simulink model "feeder_1_2_sc_lh3"  (Simulink 9.2)
settings: Solver=ode4  StartTime=0.0  StopTime=inf  FixedStep=0.0001  RelTol=1e-3
PreLoadFcn:
  | Ts=100e-6;Core_Num = 0;
PostLoadFcn:
  | Ts=100e-6;Core_Num = 0;
InitFcn:
  | Ts=100e-6;Core_Num = 0;
libraries: opal_lib x1
settings Model: ARTEMISmethode_block_infos=$$__separator__$$  Creator=DETLDAQ  LastModifiedBy=DETLDAQ
settings OptimizationCC: BlockReduction=off  BooleanDataType=off  OptimizeBlockIOStorage=off  BufferReuse=off  GlobalBufferReuse=off  ExpressionFolding=off  LocalBlockOutputs=off  OptimizeDataStoreBuffers=off  BusAssignmentInplaceUpdate=off
settings DebuggingCC: SaveWithParameterizedLinksMsg=none  SignalResolutionControl=TryResolveAllWithWarning  MultiTaskDSMMsg=warning  MultiTaskCondExecSysMsg=none  FcnCallInpInsideContextMsg=error
settings HardwareCC: TargetUnknown=on
settings RTWCC: GenCodeOnly=on
settings GRTTargetCC: CombineOutputUpdateFcns=on  GRTInterface=off
settings SimscapeCC: SimscapeNormalizeSystem=off

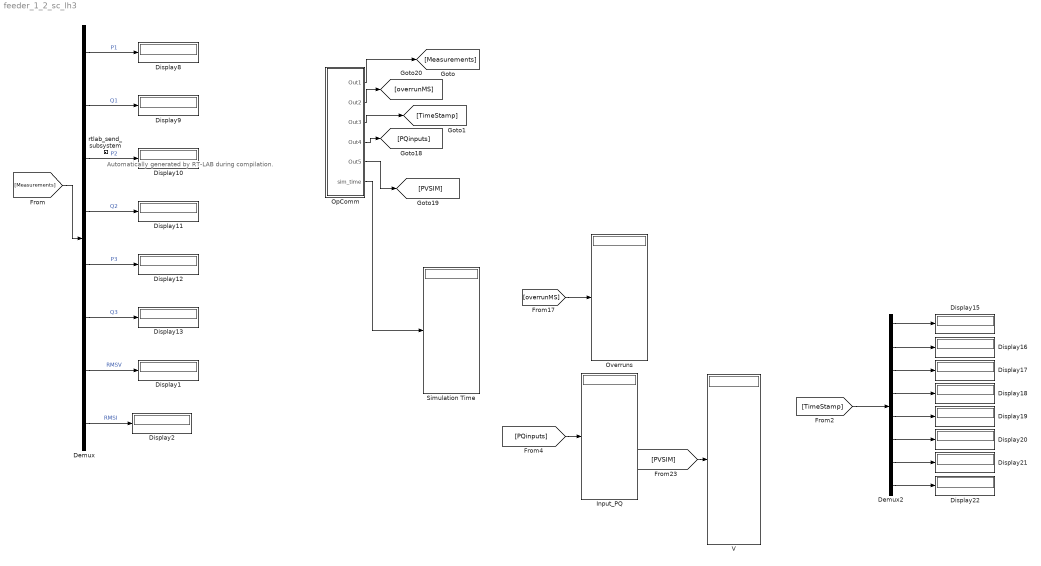
== system feeder_1_2_sc_lh3 ==
  note: Automatically generated by RT-LAB during compilation.
  Demux : Demux  Outputs=8
  Demux2 : Demux  Outputs=8
  Display{1..2,8..13,15..22} (16 alike) : Display
  Input_PQ : Display
  OpComm : Subsystem
      mask init:
      | opmaskdisplay('maskdisplay_block',gcb,'disp(''OpComm'')');
      mask Display:
      | patch([0 0.5 0.7 0],[1 1 0 0],[0.7 0.75 0.9]);
      | patch([1 0.53 0.73 1],[1 1 0 0],[1 0.8 0.7]);
      | plot([0 0 1 1 0],[0 1 1 0 0]);
      | disp('OpComm')
  Overruns : Display
  Simulation Time : Display
  V : Display
  rtlab_send_subsystem : Subsystem  Priority=-100
      mask Display: text(0,0,'');
  wires:
  Demux/7 -> Display1/1  "RMSV"
  Demux/8 -> Display2/1  "RMSI"
  OpComm/6(sim_time) -> Simulation Time/1
  OpComm/5(Out5) -> [PVSIM]
  OpComm/4(Out4) -> [PQinputs]
  [PQinputs] -> Input_PQ/1
  [PVSIM] -> V/1
  OpComm/3(Out3) -> [TimeStamp]
  OpComm/2(Out2) -> [overrunMS]
  OpComm/1(Out1) -> [Measurements]
  [overrunMS] -> Overruns/1
  Demux2/8 -> Display22/1
  Demux2/7 -> Display21/1
  Demux2/6 -> Display20/1
  Demux2/5 -> Display19/1
  Demux2/4 -> Display18/1
  Demux2/3 -> Display17/1
  Demux2/2 -> Display16/1
  Demux2/1 -> Display15/1
  [TimeStamp] -> Demux2/1
  [Measurements] -> Demux/1
  Demux/1 -> Display8/1  "P1"
  Demux/2 -> Display9/1  "Q1"
  Demux/3 -> Display10/1  "P2"
  Demux/4 -> Display11/1  "Q2"
  Demux/5 -> Display12/1  "P3"
  Demux/6 -> Display13/1  "Q3"

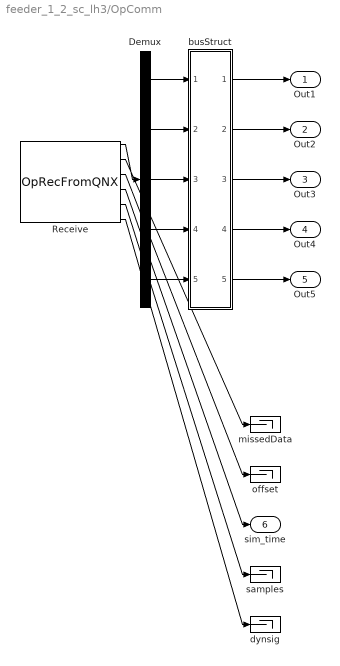
== system feeder_1_2_sc_lh3/OpComm ==
  Demux : Demux  Outputs="[8   1   8   6  12]"
  Receive : opal_lib/Communication/OpRecFromQNX  Node_num=1  Acqu_Group=1  Data_Width=35  Synchronization=on  Interpolation=on  Threshold=1.0  modelname=Feeder_1.mdl  sampletime=0.0001
  busStruct : Subsystem
  dynsig : Terminator
  missedData : Terminator
  offset : Terminator
  samples : Terminator
  Out1 : Outport
  Out2 : Outport  Port=2
  Out3 : Outport  Port=3
  Out4 : Outport  Port=4
  Out5 : Outport  Port=5
  sim_time : Outport  Port=6
  wires:
  Demux/5 -> busStruct/5(In5)
  Demux/4 -> busStruct/4(In4)
  Demux/3 -> busStruct/3(In3)
  Demux/2 -> busStruct/2(In2)
  Demux/1 -> busStruct/1(In1)
  busStruct/5(Out5) -> Out5/1
  busStruct/4(Out4) -> Out4/1
  busStruct/3(Out3) -> Out3/1
  busStruct/2(Out2) -> Out2/1
  busStruct/1(Out1) -> Out1/1
  Receive/1 -> Demux/1
  Receive/6 -> dynsig/1
  Receive/5 -> samples/1
  Receive/4 -> sim_time/1
  Receive/3 -> offset/1
  Receive/2 -> missedData/1

== system feeder_1_2_sc_lh3/rtlab_send_subsystem ==

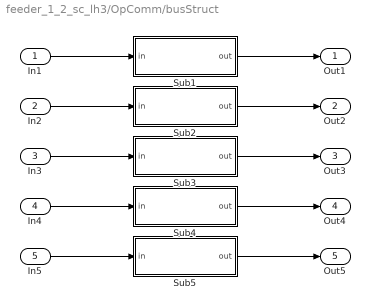
== system feeder_1_2_sc_lh3/OpComm/busStruct ==
  In1 : Inport
  In2 : Inport  Port=2
  In3 : Inport  Port=3
  In4 : Inport  Port=4
  In5 : Inport  Port=5
  Sub1 : Subsystem
  Sub2 : Subsystem
  Sub3 : Subsystem
  Sub4 : Subsystem
  Sub5 : Subsystem
  Out1 : Outport
  Out2 : Outport  Port=2
  Out3 : Outport  Port=3
  Out4 : Outport  Port=4
  Out5 : Outport  Port=5
  wires:
  Sub5/1(out) -> Out5/1
  In5/1 -> Sub5/1(in)
  Sub4/1(out) -> Out4/1
  In4/1 -> Sub4/1(in)
  Sub3/1(out) -> Out3/1
  In3/1 -> Sub3/1(in)
  Sub2/1(out) -> Out2/1
  In2/1 -> Sub2/1(in)
  Sub1/1(out) -> Out1/1
  In1/1 -> Sub1/1(in)

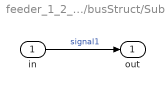
== system feeder_1_2_sc_lh3/OpComm/busStruct/Sub1 ==
  in : Inport
  out : Outport
  wires:
  in/1 -> out/1  "signal1"

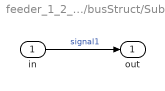
== system feeder_1_2_sc_lh3/OpComm/busStruct/Sub2 ==
  in : Inport
  out : Outport
  wires:
  in/1 -> out/1  "signal1"

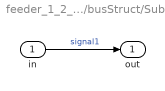
== system feeder_1_2_sc_lh3/OpComm/busStruct/Sub3 ==
  in : Inport
  out : Outport
  wires:
  in/1 -> out/1  "signal1"

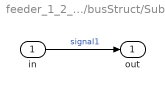
== system feeder_1_2_sc_lh3/OpComm/busStruct/Sub4 ==
  in : Inport
  out : Outport
  wires:
  in/1 -> out/1  "signal1"

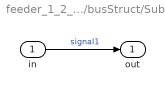
== system feeder_1_2_sc_lh3/OpComm/busStruct/Sub5 ==
  in : Inport
  out : Outport
  wires:
  in/1 -> out/1  "signal1"
